simulink model "segmentC_logic"  (R2017a)
settings: Solver=FixedStepDiscrete  StartTime=0.0  StopTime=10  FixedStep=0.01  RelTol=1e-3
PreLoadFcn:
  | robotParameters;
  | load examplePathNavigationMap.mat;
undefined symbols (not defined in the file or in its folder): axleLength, motorIp, motorSp, ticksPerRot, wheelR
libraries: mobileRoboticsTrainingLib x5, simulink_extras x1
settings Model: Creator=sseshadr  LastModifiedBy=shiremat

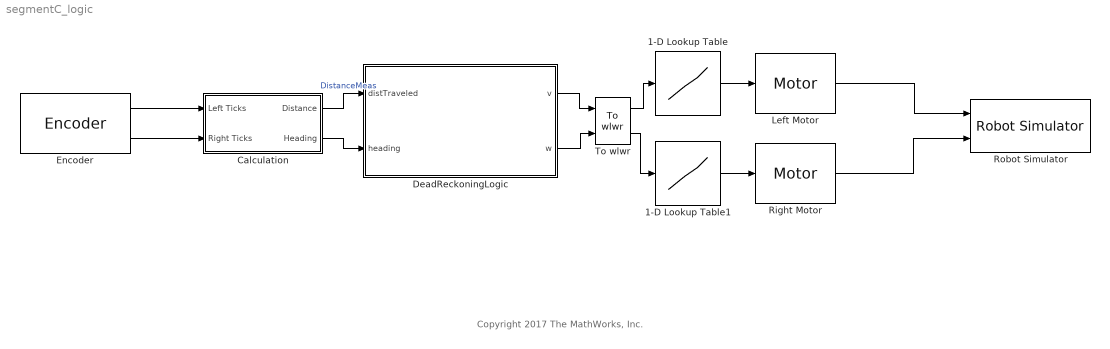
== system segmentC_logic ==
  note: Copyright 2017 The MathWorks, Inc.
  1-D Lookup Table : Lookup_n-D  NumberOfTableDimensions=1  BreakpointsForDimension1=motorSp  Table=motorIp  ExtrapMethod=Clip  InternalRulePriority=Speed  RndMeth=Simplest  InputSameDT=on
  1-D Lookup Table1 : Lookup_n-D  NumberOfTableDimensions=1  BreakpointsForDimension1=motorSp  Table=motorIp  ExtrapMethod=Clip  InternalRulePriority=Speed  RndMeth=Simplest  InputSameDT=on
  Calculation : Subsystem
  DeadReckoningLogic : Stateflow chart  TreatAsAtomicUnit=on
  Encoder : mobileRoboticsTrainingLib/Encoder  axleLength=axleLength  wheelR=wheelR  ticksPerRot=ticksPerRot
      settings: SourceProductName=Mobile Robotics Training Library
  Left Motor : mobileRoboticsTrainingLib/Motor  motorPlant=wheelMotorModel  sensorType=Speed
      settings: SourceProductName=Mobile Robotics Training Library
  Right Motor : mobileRoboticsTrainingLib/Motor  motorPlant=wheelMotorModel  sensorType=Speed
      settings: SourceProductName=Mobile Robotics Training Library
  Robot Simulator : mobileRoboticsTrainingLib/Robot Simulator  Priority=99  mapVar=mapForSim  startX=2.2772  startY=0.56625  startTheta=45  axleLength=axleLength  wheelR=wheelR
  To wlwr : mobileRoboticsTrainingLib/To wlwr  axleLength=axleLength  wheelR=wheelR
  wires:
  Calculation/1(Distance) -> DeadReckoningLogic/1(distTraveled)  "DistanceMeas"
  DeadReckoningLogic/1(v) -> To wlwr/1
  To wlwr/1 -> 1-D Lookup Table/1
  1-D Lookup Table/1 -> Left Motor/1
  1-D Lookup Table1/1 -> Right Motor/1
  Left Motor/1 -> Robot Simulator/1
  To wlwr/2 -> 1-D Lookup Table1/1
  Right Motor/1 -> Robot Simulator/2
  Encoder/1 -> Calculation/1(Left Ticks)
  Encoder/2 -> Calculation/2(Right Ticks)
  Calculation/2(Heading) -> DeadReckoningLogic/2(heading)
  DeadReckoningLogic/2(w) -> To wlwr/2

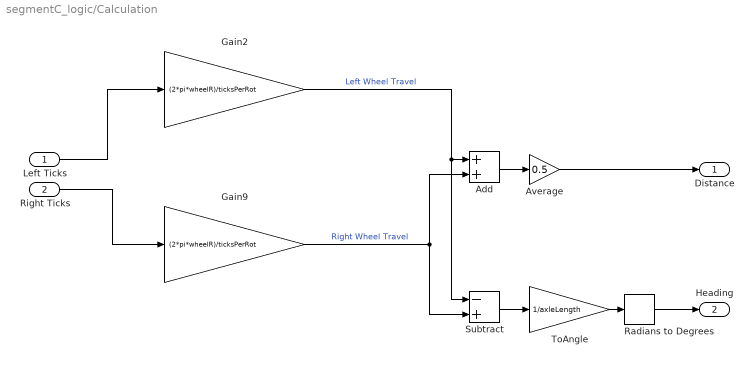
== system segmentC_logic/Calculation ==
  Left Ticks : Inport
  Right Ticks : Inport  Port=2
  Add : Sum
  Average : Gain  Gain=0.5
  Gain2 : Gain  Gain=(2*pi*wheelR)/ticksPerRot
  Gain9 : Gain  Gain=(2*pi*wheelR)/ticksPerRot
  Radians to Degrees : simulink_extras/Transformations/Radians to Degrees
  Subtract : Sum  Inputs=-+
  ToAngle : Gain  Gain=1/axleLength
  Distance : Outport
  Heading : Outport  Port=2
  wires:
  Average/1 -> Distance/1
  Add/1 -> Average/1
  Gain2/1 -> Subtract/1, Add/1  "Left Wheel Travel"
  Right Ticks/1 -> Gain9/1
  Left Ticks/1 -> Gain2/1
  Gain9/1 -> Subtract/2, Add/2  "Right Wheel Travel"
  Subtract/1 -> ToAngle/1
  ToAngle/1 -> Radians to Degrees/1
  Radians to Degrees/1 -> Heading/1

== stateflow chart segmentC_logic/DeadReckoningLogic ==
  state MoveForward
    entry:
    v = 0.5;
    currDist = distTraveled;
  state Stop
    entry:
    v = 0;
  state Rotate
    entry:
    w = 1;
    currHead = heading;
  state Stop1
    entry:
    w = 0;
  (default) -> MoveForward : %Start Dead Reckoning
  MoveForward -> Stop : [distTraveled - currDist >= 0.2]
  Stop -> Rotate
  Rotate -> Stop1 : [heading - currHead >= 45]
  data: v output; distTraveled input; heading input; w output; currDist local; currHead local
